simulink model "FINAL"  (R2021a)
settings: Solver=ode4  StartTime=0.0  StopTime=tfinal*6.5  FixedStep=dt  RelTol=1e-3
undefined symbols (not defined in the file): A, A_Lat, B, B0, B_Lat, bsi0, C, C_Lat, D, D_Lateral, Der, dt, Earth, g, K, K_D, K_Dh, K_Du, K_PI, K_PIh, K_PIu, m, mg0, p0, P_Du, P_PI, P_PIu, phi0, q0, r0, s0, sigbuilder_block, theta0, u0, v0, w0, WGS84, y, Z_Du, Z_PI, Z_PIu
libraries: simulink_extras x23, cstblocks x6, aerolibfltsims x2, shared6dof x1, aerolibtransform2 x1, aerolibasang x1, dspsigops x1
settings Model: Creator=bahbo  LastModifiedBy=bahbo

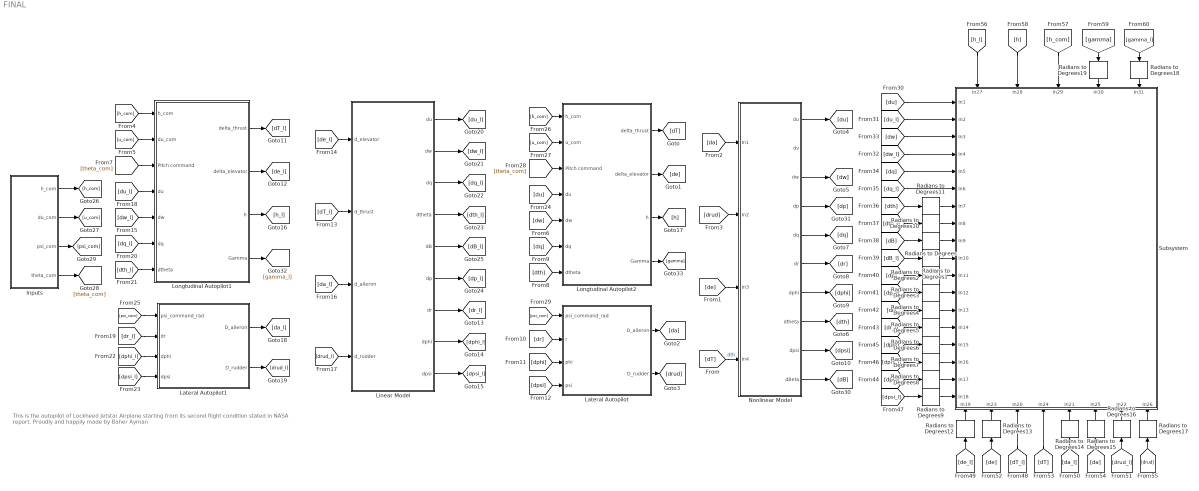
== system FINAL ==
  note: This is the autopilot of Lockheed Jetstar Airplane starting from its second flight condition stated in NASA report.
      | Proudly and happily made by Baher Ayman
  Inputs : Subsystem
  Lateral Autopilot : Subsystem
  Lateral Autopilot1 : Subsystem
  Linear Model : Subsystem
  Longtudinal Autopilot1 : Subsystem
  Longtudinal Autopilot2 : Subsystem
  Nonlinear Model : Subsystem
  Radians to Degrees{,1..19} (20 alike) : simulink_extras/Transformations/Radians to Degrees
  Subsystem : Subsystem
      settings: PortSchema="{\"entries\":[{\"content\":{\"sides\":[{\"content\":{\"connectorIds\":[\"In1\",\"In2\",\"In3\",\"In4\",\"In5\",\"In6\",\"In7\",\"In8\",\"In9\",\"In10\",\"In11\",\"In12\",\"In13\",\"In14\",\"In15\",\"In16\",\"In17\",\"In18\"]},\"type\":\"ConnectorPlacement.EquallySpacedRectSide\",\"uuid\":\"e5837911-82e8-4f0c-8622-00ee6713ee26\"},{\"content\":{\"connectorIds\":[],\"side\":\"RIGHT\"},\"type\":\"ConnectorPlacement.EquallySpacedRectSide\",\"uuid\":\"5100fd71-1e10-46a1-997f-a1a366e3eb4d\"},{\"content\":{\"connectorIds\":[\"In19\",\"In20\",\"In21\",\"In22\",\"In23\"],\"side\":\"TOP\"},\"type\":\"ConnectorPlacement.EquallySpacedRectSide\",\"uuid\":\"f99c9fc8-e14b-4975-9fcd-b405dd621b26\"},{\"content\":{\"connectorIds\":[\"In24\",\"In25\",\"In26\",\"In27\",\"In28\",\"In29\",\"In30\",\"In31\"],\"side\":\"BOTTOM\"},\"type\":\"ConnectorPlacement.EquallySpacedRectSide\",\"uuid\":\"bb89a20a-82c0-43e7-b765-f41e6636c457\"}]},\"type\":\"ConnectorPlacement.EquallySpacedConnector\",\"uuid\":\"6d5563cc-839d-4a7b-b6e3-37355380fa60\"}],\"packageUris\":[\"http://schema.mathworks.com/mf0/Connector/R2020b\"],\"version\":\"1.0\"}"
  wires:
  [de] -> Nonlinear Model/3(In3)
  Longtudinal Autopilot2/2(delta_elevator) -> [de]
  Lateral Autopilot/2(D_rudder) -> [drud]
  [drud] -> Nonlinear Model/2(In2)
  Nonlinear Model/5(dq) -> [dq]
  Nonlinear Model/8(dtheta) -> [dth]
  [dpsi] -> Lateral Autopilot/4(psi)
  Nonlinear Model/6(dr) -> [dr]
  [dq] -> Longtudinal Autopilot2/6(dq)
  Nonlinear Model/9(dpsi) -> [dpsi]
  Nonlinear Model/1(du) -> [du]
  Lateral Autopilot/1(D_aileron) -> [da]
  Nonlinear Model/7(dphi) -> [dphi]
  [dT] -> Nonlinear Model/4(In4)  "dth"
  [da] -> Nonlinear Model/1(In1)
  Longtudinal Autopilot2/1(delta_thrust) -> [dT]
  Nonlinear Model/3(dw) -> [dw]
  [dphi] -> Lateral Autopilot/3(phi)
  [dth] -> Longtudinal Autopilot2/7(dtheta)
  [dr] -> Lateral Autopilot/2(r)
  Linear Model/1(du) -> [du_l]
  Linear Model/7(dr) -> [dr_l]
  Linear Model/3(dq) -> [dq_l]
  Longtudinal Autopilot1/3(h) -> [h_l]
  [dpsi_l] -> Lateral Autopilot1/4(dpsi)
  [dw_l] -> Longtudinal Autopilot1/5(dw)
  Linear Model/9(dpsi) -> [dpsi_l]
  Longtudinal Autopilot1/1(delta_thrust) -> [dT_l]
  Lateral Autopilot1/2(D_rudder) -> [drud_l]
  [dphi_l] -> Lateral Autopilot1/3(dphi)
  [drud_l] -> Linear Model/4(d_rudder)
  [dq_l] -> Longtudinal Autopilot1/6(dq)
  [de_l] -> Linear Model/1(d_elevator)
  [du_l] -> Longtudinal Autopilot1/4(du)
  Linear Model/5(dB) -> [dB_l]
  Linear Model/6(dp) -> [dp_l]
  [da_l] -> Linear Model/3(d_aileron)
  Longtudinal Autopilot1/2(delta_elevator) -> [de_l]
  Lateral Autopilot1/1(D_aileron) -> [da_l]
  Linear Model/4(dtheta) -> [dth_l]
  [dT_l] -> Linear Model/2(d_thrust)
  [dr_l] -> Lateral Autopilot1/2(dr)
  [dth_l] -> Longtudinal Autopilot1/7(dtheta)
  Linear Model/8(dphi) -> [dphi_l]
  Linear Model/2(dw) -> [dw_l]
  [du] -> Longtudinal Autopilot2/4(du)
  [dw] -> Longtudinal Autopilot2/5(dw)
  Inputs/2(du_com) -> [u_com]
  Inputs/4(theta_com) -> [theta_com]
  Inputs/1(h_com) -> [h_com]
  Inputs/3(psi_com) -> [psi_com]
  [h_com] -> Longtudinal Autopilot1/1(h_com)
  [u_com] -> Longtudinal Autopilot1/2(du_com)
  [theta_com] -> Longtudinal Autopilot1/3(Pitch command)
  [psi_com] -> Lateral Autopilot1/1(psi_command_rad)
  [h_com] -> Longtudinal Autopilot2/1(h_com)
  [u_com] -> Longtudinal Autopilot2/2(u_com)
  [theta_com] -> Longtudinal Autopilot2/3(Pitch command)
  [psi_com] -> Lateral Autopilot/1(psi_command_rad)
  Nonlinear Model/10(dBeta) -> [dB]
  [du] -> Subsystem/1(In1)
  [du_l] -> Subsystem/2(In2)
  [dw_l] -> Subsystem/4(In4)
  [dw] -> Subsystem/3(In3)
  [dq] -> Subsystem/5(In5)
  [dq_l] -> Subsystem/6(In6)
  Nonlinear Model/4(dp) -> [dp]
  [dT_l] -> Subsystem/26(In20)
  [dT] -> Subsystem/27(In24)
  Longtudinal Autopilot2/3(h) -> [h]
  [h_l] -> Subsystem/19(In27)
  [h] -> Subsystem/20(In28)
  [h_com] -> Subsystem/21(In29)
  Radians to Degrees9/1 -> Subsystem/18(In18)
  [dpsi_l] -> Radians to Degrees9/1
  [dpsi] -> Radians to Degrees8/1
  Radians to Degrees8/1 -> Subsystem/17(In17)
  [dphi_l] -> Radians to Degrees7/1
  Radians to Degrees7/1 -> Subsystem/16(In16)
  [dphi] -> Radians to Degrees6/1
  Radians to Degrees6/1 -> Subsystem/15(In15)
  [dr_l] -> Radians to Degrees5/1
  Radians to Degrees5/1 -> Subsystem/14(In14)
  [dr] -> Radians to Degrees4/1
  Radians to Degrees4/1 -> Subsystem/13(In13)
  [dp_l] -> Radians to Degrees3/1
  Radians to Degrees3/1 -> Subsystem/12(In12)
  [dp] -> Radians to Degrees2/1
  Radians to Degrees2/1 -> Subsystem/11(In11)
  [dB_l] -> Radians to Degrees1/1
  Radians to Degrees1/1 -> Subsystem/10(In10)
  [dB] -> Radians to Degrees/1
  Radians to Degrees/1 -> Subsystem/9(In9)
  [dth] -> Radians to Degrees11/1
  Radians to Degrees11/1 -> Subsystem/7(In7)
  [dth_l] -> Radians to Degrees10/1
  Radians to Degrees10/1 -> Subsystem/8(In8)
  Radians to Degrees16/1 -> Subsystem/30(In22)
  [drud_l] -> Radians to Degrees16/1
  [drud] -> Radians to Degrees17/1
  Radians to Degrees17/1 -> Subsystem/31(In26)
  [da] -> Radians to Degrees15/1
  Radians to Degrees15/1 -> Subsystem/29(In25)
  [da_l] -> Radians to Degrees14/1
  Radians to Degrees14/1 -> Subsystem/28(In21)
  [de] -> Radians to Degrees13/1
  Radians to Degrees13/1 -> Subsystem/25(In23)
  [de_l] -> Radians to Degrees12/1
  Radians to Degrees12/1 -> Subsystem/24(In19)
  Longtudinal Autopilot1/4(Gamma) -> [gamma_l]
  Longtudinal Autopilot2/4(Gamma) -> [gamma]
  [gamma] -> Radians to Degrees19/1
  [gamma_l] -> Radians to Degrees18/1
  Radians to Degrees18/1 -> Subsystem/23(In31)
  Radians to Degrees19/1 -> Subsystem/22(In30)

== system FINAL/Inputs ==
  Constant : Constant  Commented=on  Value=12
  Degrees to Radians : simulink_extras/Transformations/Degrees to Radians  Commented=on
  Inputs Signals : Subsystem  Tag=STV Subsys  LoadFcn=sigbuilder_block('load');  StartFcn=sigbuilder_block('start');  StopFcn=sigbuilder_block('stop');  ClipboardFcn=sigbuilder_block('clipboard');  mask(Sigbuilder block){tuvar=[0:10]}
      mask help: Simulink:masks:SigbuilderBlock_MD
      mask init:
      | if ~strcmp(get_param(bdroot(gcbh),'SimulationStatus'),'stopped') tuvar = sigbuilder_block('maskInit'); end
      settings: CopyFcn=sigbuilder_block('copy');  DeleteFcn=sigbuilder_block('delete');  ModelCloseFcn=sigbuilder_block('modelClose');  PreSaveFcn=sigbuilder_block('preSave');  PauseFcn=sigbuilder_block('pause');  ContinueFcn=sigbuilder_block('continue');  NameChangeFcn=sigbuilder_block('namechange');  OpenFcn=sigbuilder_block('open',[6 33 1012.5 444 ]);  CloseFcn=sigbuilder_block('close');
      mask Display: plot(0, 0, 100, 100,[2, 2, 32, 32, 2], [68, 8, 8, 68, 68],[32, 2], [38, 38], [32, 19, 2],[53, 60, 44], [32, 17, 17, 2],[16, 16, 31, 31]);txt = getActiveGroup(gcbh);text(2, 100, txt,'verticalAlignment', 'top');
  h_com : Outport
  du_com : Outport  Port=2
  psi_com : Outport  Port=3
  theta_com : Outport  Port=4
  wires:
  Inputs Signals/3(Velocity Com.) -> du_com/1
  Constant/1 -> Degrees to Radians/1
  Degrees to Radians/1 -> theta_com/1
  Inputs Signals/1(Altitude Command) -> h_com/1
  Inputs Signals/2(Psi Command) -> psi_com/1

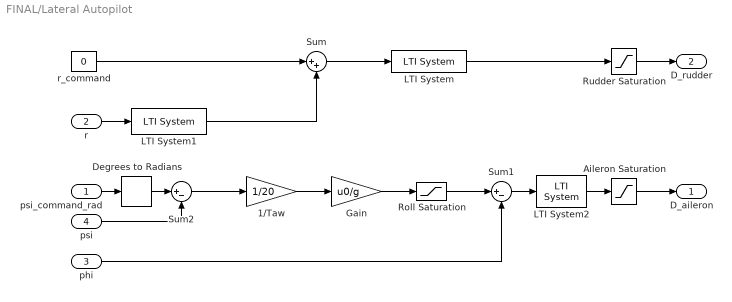
== system FINAL/Lateral Autopilot ==
  psi_command_rad : Inport
  r : Inport  Port=2
  phi : Inport  Port=3
  psi : Inport  Port=4
  1/Taw : Gain  Gain=1/20
  Aileron Saturation : Saturate  UpperLimit=50*pi/180  LowerLimit=-50*pi/180
  Degrees to Radians : simulink_extras/Transformations/Degrees to Radians
  Gain : Gain  Gain=u0/g
  LTI System : cstblocks/LTI System  sys=servo  IC=[]
  LTI System1 : cstblocks/LTI System  sys=yaw_damper  IC=[]
  LTI System2 : cstblocks/LTI System  sys=roll_ctrl  IC=[]
  Roll Saturation : Saturate  UpperLimit=30*pi/180  LowerLimit=-30*pi/180
  Rudder Saturation : Saturate  UpperLimit=15*pi/180  LowerLimit=-15*pi/180
  Sum : Sum  Inputs=|++
  Sum1 : Sum  Inputs=|+-
  Sum2 : Sum  Inputs=|+-
  r_command : Constant  Value=0
  D_aileron : Outport
  D_rudder : Outport  Port=2
  wires:
  Sum2/1 -> 1/Taw/1
  Sum/1 -> LTI System/1
  r/1 -> LTI System1/1
  Rudder Saturation/1 -> D_rudder/1
  Roll Saturation/1 -> Sum1/1
  Aileron Saturation/1 -> D_aileron/1
  r_command/1 -> Sum/1
  phi/1 -> Sum1/2
  psi/1 -> Sum2/2
  LTI System1/1 -> Sum/2
  LTI System/1 -> Rudder Saturation/1
  Sum1/1 -> LTI System2/1
  1/Taw/1 -> Gain/1
  Gain/1 -> Roll Saturation/1
  LTI System2/1 -> Aileron Saturation/1
  psi_command_rad/1 -> Degrees to Radians/1
  Degrees to Radians/1 -> Sum2/1

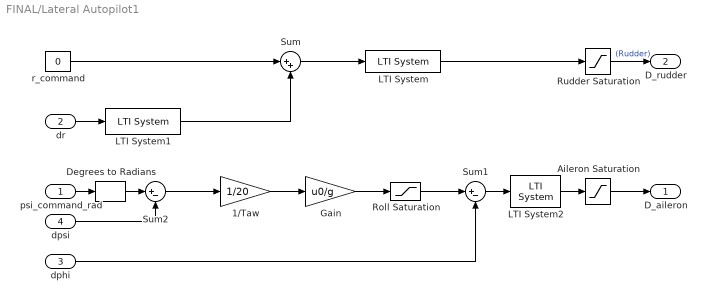
== system FINAL/Lateral Autopilot1 ==
  psi_command_rad : Inport
  dr : Inport  Port=2
  dphi : Inport  Port=3
  dpsi : Inport  Port=4
  1/Taw : Gain  Gain=1/20
  Aileron Saturation : Saturate  UpperLimit=50*pi/180  LowerLimit=-50*pi/180
  Degrees to Radians : simulink_extras/Transformations/Degrees to Radians
  Gain : Gain  Gain=u0/g
  LTI System : cstblocks/LTI System  sys=servo  IC=[]
  LTI System1 : cstblocks/LTI System  sys=yaw_damper  IC=[]
  LTI System2 : cstblocks/LTI System  sys=roll_ctrl  IC=[]
  Roll Saturation : Saturate  UpperLimit=30*pi/180  LowerLimit=-30*pi/180
  Rudder Saturation : Saturate  UpperLimit=15*pi/180  LowerLimit=-15*pi/180
  Sum : Sum  Inputs=|++
  Sum1 : Sum  Inputs=|+-
  Sum2 : Sum  Inputs=|+-
  r_command : Constant  Value=0
  D_aileron : Outport
  D_rudder : Outport  Port=2
  wires:
  Sum2/1 -> 1/Taw/1
  Sum/1 -> LTI System/1
  dr/1 -> LTI System1/1
  Rudder Saturation/1 -> D_rudder/1  "(Rudder)"
  Roll Saturation/1 -> Sum1/1
  Aileron Saturation/1 -> D_aileron/1
  r_command/1 -> Sum/1
  dphi/1 -> Sum1/2
  dpsi/1 -> Sum2/2
  LTI System1/1 -> Sum/2
  LTI System/1 -> Rudder Saturation/1
  Sum1/1 -> LTI System2/1
  1/Taw/1 -> Gain/1
  Gain/1 -> Roll Saturation/1
  LTI System2/1 -> Aileron Saturation/1
  psi_command_rad/1 -> Degrees to Radians/1
  Degrees to Radians/1 -> Sum2/1

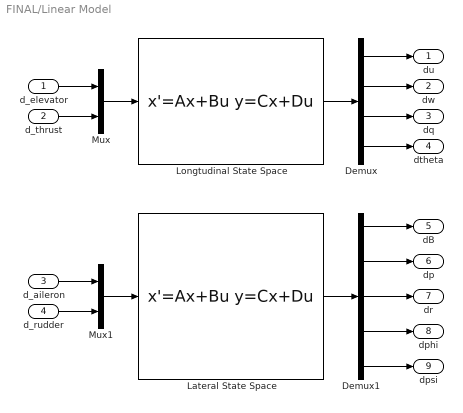
== system FINAL/Linear Model ==
  d_elevator : Inport
  d_thrust : Inport  Port=2
  d_aileron : Inport  Port=3
  d_rudder : Inport  Port=4
  Demux : Demux
  Demux1 : Demux  Outputs=5
  Lateral State Space : StateSpace  A=A_Lat  B=B_Lat  C=C_Lat  D=D_Lateral  InitialCondition=0
  Longtudinal State Space : StateSpace  A=A  B=B  C=C  D=D  InitialCondition=0
  Mux : Mux  Inputs=2
  Mux1 : Mux  Inputs=2
  du : Outport
  dw : Outport  Port=2
  dq : Outport  Port=3
  dtheta : Outport  Port=4
  dB : Outport  Port=5
  dp : Outport  Port=6
  dr : Outport  Port=7
  dphi : Outport  Port=8
  dpsi : Outport  Port=9
  wires:
  Demux/3 -> dq/1
  Lateral State Space/1 -> Demux1/1
  Demux1/4 -> dphi/1
  d_elevator/1 -> Mux/1
  Demux/4 -> dtheta/1
  Mux/1 -> Longtudinal State Space/1
  Mux1/1 -> Lateral State Space/1
  d_thrust/1 -> Mux/2
  Demux1/5 -> dpsi/1
  Demux1/1 -> dB/1
  Demux1/2 -> dp/1
  Demux/2 -> dw/1
  d_aileron/1 -> Mux1/1
  Demux/1 -> du/1
  Demux1/3 -> dr/1
  Longtudinal State Space/1 -> Demux/1
  d_rudder/1 -> Mux1/2

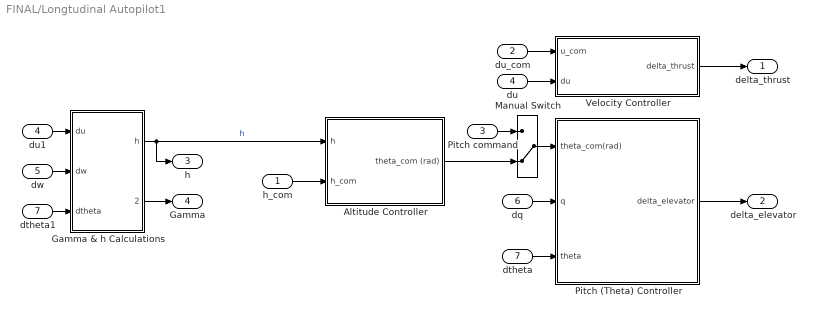
== system FINAL/Longtudinal Autopilot1 ==
  h_com : Inport
  du_com : Inport  Port=2
  Pitch command : Inport  Port=3
  du : Inport  Port=4
  dw : Inport  Port=5
  dq : Inport  Port=6
  dtheta : Inport  Port=7
  Altitude Controller : Subsystem
  Gamma & h Calculations : Subsystem
  Manual Switch : ManualSwitch  CurrentSetting=0
  Pitch (Theta) Controller : Subsystem
  Velocity Controller : Subsystem
  dtheta1 : InportShadow  Port=7
  du1 : InportShadow  Port=4
  delta_thrust : Outport
  delta_elevator : Outport  Port=2
  h : Outport  Port=3
  Gamma : Outport  Port=4
  wires:
  du/1 -> Velocity Controller/2(du)
  Velocity Controller/1(delta_thrust) -> delta_thrust/1
  dtheta/1 -> Pitch (Theta) Controller/3(theta)
  h_com/1 -> Altitude Controller/2(h_com)
  du_com/1 -> Velocity Controller/1(u_com)
  Pitch (Theta) Controller/1(delta_elevator) -> delta_elevator/1
  dq/1 -> Pitch (Theta) Controller/2(q)
  Altitude Controller/1(theta_com (rad)) -> Manual Switch/2
  Manual Switch/1 -> Pitch (Theta) Controller/1(theta_com(rad))
  Pitch command/1 -> Manual Switch/1
  du1/1 -> Gamma & h Calculations/1(du)
  dtheta1/1 -> Gamma & h Calculations/3(dtheta)
  Gamma & h Calculations/1(h) -> Altitude Controller/1(h), h/1  "h"
  dw/1 -> Gamma & h Calculations/2(dw)
  Gamma & h Calculations/2(gamma) -> Gamma/1

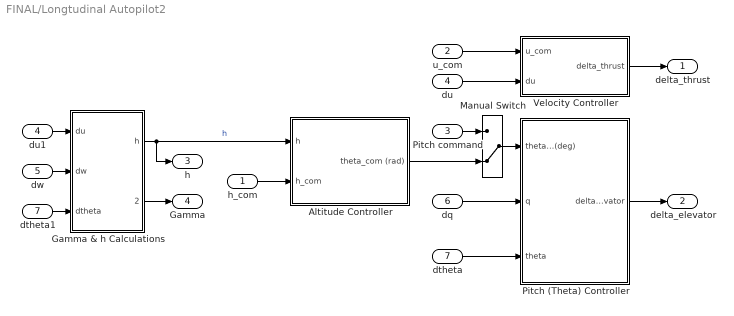
== system FINAL/Longtudinal Autopilot2 ==
  h_com : Inport
  u_com : Inport  Port=2
  Pitch command : Inport  Port=3
  du : Inport  Port=4
  dw : Inport  Port=5
  dq : Inport  Port=6
  dtheta : Inport  Port=7
  Altitude Controller : Subsystem
  Gamma & h Calculations : Subsystem
  Manual Switch : ManualSwitch  CurrentSetting=0
  Pitch (Theta) Controller : Subsystem
  Velocity Controller : Subsystem
  dtheta1 : InportShadow  Port=7
  du1 : InportShadow  Port=4
  delta_thrust : Outport
  delta_elevator : Outport  Port=2
  h : Outport  Port=3
  Gamma : Outport  Port=4
  wires:
  du/1 -> Velocity Controller/2(du)
  Velocity Controller/1(delta_thrust) -> delta_thrust/1
  dtheta/1 -> Pitch (Theta) Controller/3(theta)
  h_com/1 -> Altitude Controller/2(h_com)
  u_com/1 -> Velocity Controller/1(u_com)
  Pitch (Theta) Controller/1(delta_elevator) -> delta_elevator/1
  dq/1 -> Pitch (Theta) Controller/2(q)
  Altitude Controller/1(theta_com (rad)) -> Manual Switch/2
  Manual Switch/1 -> Pitch (Theta) Controller/1(theta_com(deg))
  Pitch command/1 -> Manual Switch/1
  du1/1 -> Gamma & h Calculations/1(du)
  dtheta1/1 -> Gamma & h Calculations/3(dtheta)
  Gamma & h Calculations/1(h) -> Altitude Controller/1(h), h/1  "h"
  dw/1 -> Gamma & h Calculations/2(dw)
  Gamma & h Calculations/2(gamma) -> Gamma/1

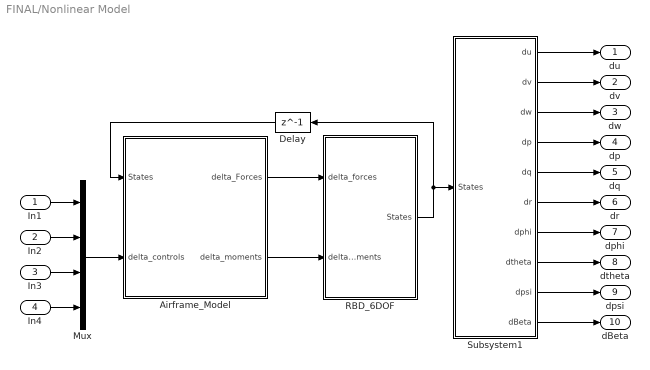
== system FINAL/Nonlinear Model ==
  In1 : Inport
  In2 : Inport  Port=2
  In3 : Inport  Port=3
  In4 : Inport  Port=4
  Airframe_Model : Subsystem
  Delay : Delay  DelayLength=1  InitialCondition=K
  Mux : Mux
  RBD_6DOF : Subsystem
  Subsystem1 : Subsystem
  du : Outport
  dv : Outport  Port=2
  dw : Outport  Port=3
  dp : Outport  Port=4
  dq : Outport  Port=5
  dr : Outport  Port=6
  dphi : Outport  Port=7
  dtheta : Outport  Port=8
  dpsi : Outport  Port=9
  dBeta : Outport  Port=10
  wires:
  RBD_6DOF/1(States) -> Delay/1, Subsystem1/1(States)
  Airframe_Model/2(delta_moments) -> RBD_6DOF/2(delta_moments)
  Subsystem1/4(dp) -> dp/1
  Delay/1 -> Airframe_Model/1(States)
  Subsystem1/7(dphi) -> dphi/1
  Mux/1 -> Airframe_Model/2(delta_controls)
  In2/1 -> Mux/2
  Airframe_Model/1(delta_Forces) -> RBD_6DOF/1(delta_forces)
  Subsystem1/8(dtheta) -> dtheta/1
  In1/1 -> Mux/1
  Subsystem1/6(dr) -> dr/1
  Subsystem1/5(dq) -> dq/1
  In3/1 -> Mux/3
  Subsystem1/1(du) -> du/1
  In4/1 -> Mux/4
  Subsystem1/3(dw) -> dw/1
  Subsystem1/10(dBeta) -> dBeta/1
  Subsystem1/9(dpsi) -> dpsi/1
  Subsystem1/2(dv) -> dv/1

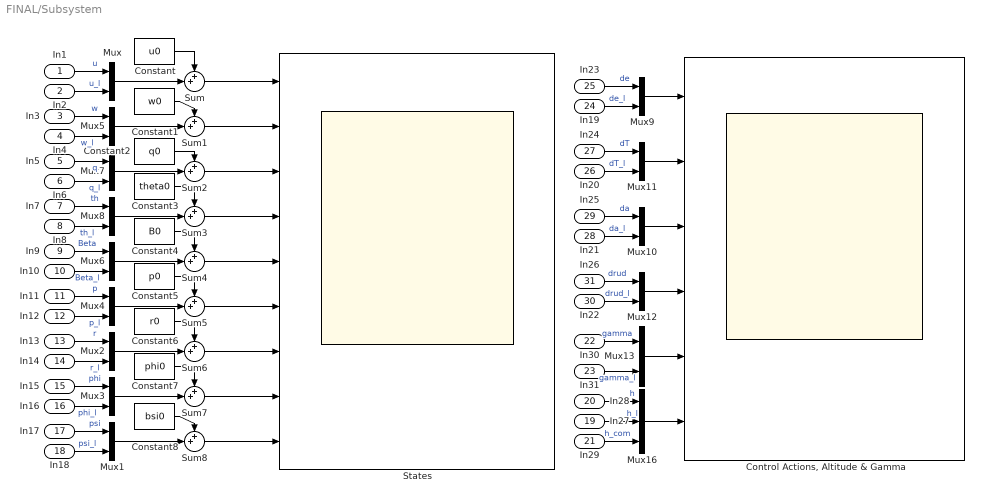
== system FINAL/Subsystem ==
  In1 : Inport
  In2 : Inport  Port=2
  In3 : Inport  Port=3
  In4 : Inport  Port=4
  In5 : Inport  Port=5
  In6 : Inport  Port=6
  In7 : Inport  Port=7
  In8 : Inport  Port=8
  In9 : Inport  Port=9
  In10 : Inport  Port=10
  In11 : Inport  Port=11
  In12 : Inport  Port=12
  In13 : Inport  Port=13
  In14 : Inport  Port=14
  In15 : Inport  Port=15
  In16 : Inport  Port=16
  In17 : Inport  Port=17
  In18 : Inport  Port=18
  In27 : Inport  Port=19
  In28 : Inport  Port=20
  In29 : Inport  Port=21
  In30 : Inport  Port=22
  In31 : Inport  Port=23
  In19 : Inport  Port=24
  In23 : Inport  Port=25
  In20 : Inport  Port=26
  In24 : Inport  Port=27
  In21 : Inport  Port=28
  In25 : Inport  Port=29
  In22 : Inport  Port=30
  In26 : Inport  Port=31
  Constant : Constant  Value=u0
  Constant1 : Constant  Value=w0
  Constant2 : Constant  Value=q0
  Constant3 : Constant  Value=theta0
  Constant4 : Constant  Value=B0
  Constant5 : Constant  Value=p0
  Constant6 : Constant  Value=r0
  Constant7 : Constant  Value=phi0
  Constant8 : Constant  Value=bsi0
  "Control Actions, Altitude & Gamma" : Scope  NumInputPorts=6
  Mux{,1..13} (14 alike) : Mux  Inputs=2
  Mux16 : Mux  Inputs=3
  States : Scope  NumInputPorts=9
  Sum{,1..8} (9 alike) : Sum  Inputs=++|
  wires:
  Mux9/1 -> "Control Actions, Altitude & Gamma"/1
  Mux10/1 -> "Control Actions, Altitude & Gamma"/3
  Mux11/1 -> "Control Actions, Altitude & Gamma"/2
  Mux12/1 -> "Control Actions, Altitude & Gamma"/4
  Mux16/1 -> "Control Actions, Altitude & Gamma"/6
  In1/1 -> Mux/1  "u"
  In3/1 -> Mux5/1  "w"
  In4/1 -> Mux5/2  "w_l"
  In5/1 -> Mux7/1  "q"
  In6/1 -> Mux7/2  "q_l"
  In7/1 -> Mux8/1  "th"
  In8/1 -> Mux8/2  "th_l"
  In9/1 -> Mux6/1  "Beta"
  In10/1 -> Mux6/2  "Beta_l"
  In11/1 -> Mux4/1  "p"
  In12/1 -> Mux4/2  "p_l"
  In13/1 -> Mux2/1  "r"
  In14/1 -> Mux2/2  "r_l"
  In15/1 -> Mux3/1  "phi"
  In16/1 -> Mux3/2  "phi_l"
  In17/1 -> Mux1/1  "psi"
  In18/1 -> Mux1/2  "psi_l"
  In2/1 -> Mux/2  "u_l"
  In19/1 -> Mux9/2  "de_l"
  In20/1 -> Mux11/2  "dT_l"
  In21/1 -> Mux10/2  "da_l"
  In22/1 -> Mux12/2  "drud_l"
  In23/1 -> Mux9/1  "de"
  In24/1 -> Mux11/1  "dT"
  In25/1 -> Mux10/1  "da"
  In26/1 -> Mux12/1  "drud"
  In27/1 -> Mux16/2  "h_l"
  In28/1 -> Mux16/1  "h"
  In29/1 -> Mux16/3  "h_com"
  In30/1 -> Mux13/1  "gamma"
  In31/1 -> Mux13/2  "gamma_l"
  Mux13/1 -> "Control Actions, Altitude & Gamma"/5
  Sum/1 -> States/1
  Mux/1 -> Sum/2
  Constant/1 -> Sum/1
  Constant1/1 -> Sum1/1
  Mux5/1 -> Sum1/2
  Sum1/1 -> States/2
  Constant2/1 -> Sum2/1
  Mux7/1 -> Sum2/2
  Sum2/1 -> States/3
  Constant3/1 -> Sum3/1
  Mux8/1 -> Sum3/2
  Sum3/1 -> States/4
  Constant4/1 -> Sum4/1
  Mux6/1 -> Sum4/2
  Sum4/1 -> States/5
  Constant5/1 -> Sum5/1
  Mux4/1 -> Sum5/2
  Sum5/1 -> States/6
  Constant6/1 -> Sum6/1
  Mux2/1 -> Sum6/2
  Sum6/1 -> States/7
  Constant7/1 -> Sum7/1
  Mux3/1 -> Sum7/2
  Sum7/1 -> States/8
  Constant8/1 -> Sum8/1
  Mux1/1 -> Sum8/2
  Sum8/1 -> States/9

== system FINAL/Inputs/Inputs Signals ==
  Demux : Demux  Tag=STV Demux  Outputs=3
      settings: DisplayOption=none
  FromWs : FromWorkspace  Tag=STV FromWs  VariableName=tuvar
      SigBuilderData=|
      | common.afterFinalStr = 'Extrapolate'
      | common.sampleTime = 0
      | dataSet.timeRange = [0 1300]
      | dataSet.name = 'Group 1'
      | sbobj.Groups.Name = 'Group 1'
      | sbobj.Groups.Signals(1).Name = 'Altitude Command'
      | sbobj.Groups.Signals(1).XData = [0 400 520 760 760 880 1284 1300]
      | sbobj.Groups.Signals(1).YData = [0 10000 10000 10000 10100 10100 0 0]
      | sbobj.Groups.Signals(2).Name = 'Psi Command'
      | sbobj.Groups.Signals(2).XData = [0 520 520 760 760 1300]
      | sbobj.Groups.Signals(2).YData = [0 0 360 360 390 390]
      | sbobj.Groups.Signals(3).Name = 'Velocity Com.'
      | sbobj.Groups.Signals(3).XData = [0 400 1000 1284 1300]
      | sbobj.Groups.Signals(3).YData = [0 400 400 0 0]
      | sbobj.Groups.TimeRange = [0 1300]
  Altitude Command : Outport  Tag=STV Outport
  Psi Command : Outport  Tag=STV Outport  Port=2
  Velocity Com. : Outport  Tag=STV Outport  Port=3
  wires:
  FromWs/1 -> Demux/1
  Demux/1 -> Altitude Command/1
  Demux/2 -> Psi Command/1
  Demux/3 -> Velocity Com./1

== system FINAL/Longtudinal Autopilot1/Altitude Controller ==
  note: Altitude Controller
  h : Inport
  h_com : Inport  Port=2
  Differentiator : Derivative
  Kd : Gain  Gain=K_Dh
  Kp : Gain  Gain=K_PIh
  Sum : Sum  Inputs=|+-
  Sum1 : Sum  Inputs=|+-
  theta_com (rad) : Outport
  wires:
  Sum/1 -> theta_com (rad)/1
  Sum1/1 -> Kp/1
  Kd/1 -> Sum/2
  h_com/1 -> Sum1/1
  Kp/1 -> Sum/1
  Differentiator/1 -> Kd/1
  h/1 -> Sum1/2, Differentiator/1

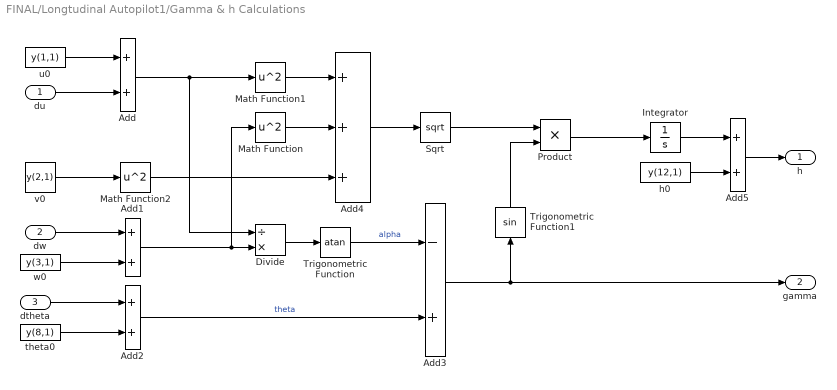
== system FINAL/Longtudinal Autopilot1/Gamma & h Calculations ==
  du : Inport
  dw : Inport  Port=2
  dtheta : Inport  Port=3
  Add{,1..2,5} (4 alike) : Sum
  Add3 : Sum  Inputs=-+
  Add4 : Sum  Inputs=+++
  Divide : Product  Inputs=/*
  Integrator : Integrator
  Math Function : Math  Operator=square  SignedPower=on  SaturateOnIntegerOverflow=on
  Math Function1 : Math  Operator=square  SignedPower=on  SaturateOnIntegerOverflow=on
  Math Function2 : Math  Operator=square  SignedPower=on  SaturateOnIntegerOverflow=on
  Product : Product
  Sqrt : Sqrt  SaturateOnIntegerOverflow=on
  Trigonometric Function : Trigonometry  Operator=atan
  Trigonometric Function1 : Trigonometry
  h0 : Constant  Value=y(12,1)
  theta0 : Constant  Value=y(8,1)
  u0 : Constant  Value=y(1,1)
  v0 : Constant  Value=y(2,1)
  w0 : Constant  Value=y(3,1)
  h : Outport
  gamma : Outport  Port=2
  wires:
  Integrator/1 -> Add5/1
  Product/1 -> Integrator/1
  h0/1 -> Add5/2
  Divide/1 -> Trigonometric Function/1
  Math Function1/1 -> Add4/1
  Add5/1 -> h/1
  Trigonometric Function1/1 -> Product/2
  Add3/1 -> gamma/1, Trigonometric Function1/1
  Add4/1 -> Sqrt/1
  Trigonometric Function/1 -> Add3/1  "alpha"
  Math Function/1 -> Add4/2
  Sqrt/1 -> Product/1
  Math Function2/1 -> Add4/3
  v0/1 -> Math Function2/1
  Add/1 -> Math Function1/1, Divide/1
  u0/1 -> Add/1
  du/1 -> Add/2
  w0/1 -> Add1/2
  dw/1 -> Add1/1
  Add1/1 -> Math Function/1, Divide/2
  dtheta/1 -> Add2/1
  theta0/1 -> Add2/2
  Add2/1 -> Add3/2  "theta"

== system FINAL/Longtudinal Autopilot1/Pitch (Theta) Controller ==
  note: Pitch Controller
  theta_com(rad) : Inport
  q : Inport  Port=2
  theta : Inport  Port=3
  Elevator Saturation : Saturate  UpperLimit=25*pi/180  LowerLimit=-25*pi/180
  Kd : Gain  Gain=K_D
  Sum : Sum  Inputs=|+-
  Sum1 : Sum  Inputs=|+-
  Zero-Pole : ZeroPole  Zeros=[Z_PI]  Poles=[P_PI]  Gain=[K_PI]
  servo : TransferFcn  Numerator=[-10]  Denominator=[1 10]
  delta_elevator : Outport
  wires:
  q/1 -> Kd/1
  Zero-Pole/1 -> Sum/1
  Sum/1 -> servo/1
  theta_com(rad)/1 -> Sum1/1
  Kd/1 -> Sum/2
  theta/1 -> Sum1/2
  servo/1 -> Elevator Saturation/1
  Sum1/1 -> Zero-Pole/1
  Elevator Saturation/1 -> delta_elevator/1

== system FINAL/Longtudinal Autopilot1/Velocity Controller ==
  note: Velocity Controller
  u_com : Inport
  du : Inport  Port=2
  Engine Saturation : Saturate  UpperLimit=3*3700  LowerLimit=-1500
  Sum : Sum  Inputs=|+-
  Sum1 : Sum  Inputs=|+-
  Zero-Pole : ZeroPole  Zeros=[Z_Du]  Poles=[P_Du]  Gain=[K_Du]
  Zero-Pole1 : ZeroPole  Zeros=[Z_PIu]  Poles=[P_PIu]  Gain=[K_PIu]
  engine_timelag : TransferFcn  Numerator=[0.1]  Denominator=[1 0.1]
  servo : TransferFcn  Numerator=[10]  Denominator=[1 10]
  delta_thrust : Outport
  wires:
  u_com/1 -> Sum1/1
  Sum/1 -> servo/1
  servo/1 -> engine_timelag/1
  du/1 -> Sum1/2, Zero-Pole/1
  engine_timelag/1 -> Engine Saturation/1
  Zero-Pole/1 -> Sum/2
  Sum1/1 -> Zero-Pole1/1
  Zero-Pole1/1 -> Sum/1
  Engine Saturation/1 -> delta_thrust/1

== system FINAL/Longtudinal Autopilot2/Altitude Controller ==
  note: Altitude Controller
  h : Inport
  h_com : Inport  Port=2
  Differentiator : Derivative
  Kd : Gain  Gain=K_Dh
  Kp : Gain  Gain=K_PIh
  Sum : Sum  Inputs=|+-
  Sum1 : Sum  Inputs=|+-
  theta_com (rad) : Outport
  wires:
  Sum/1 -> theta_com (rad)/1
  Sum1/1 -> Kp/1
  Kd/1 -> Sum/2
  h_com/1 -> Sum1/1
  Kp/1 -> Sum/1
  Differentiator/1 -> Kd/1
  h/1 -> Sum1/2, Differentiator/1

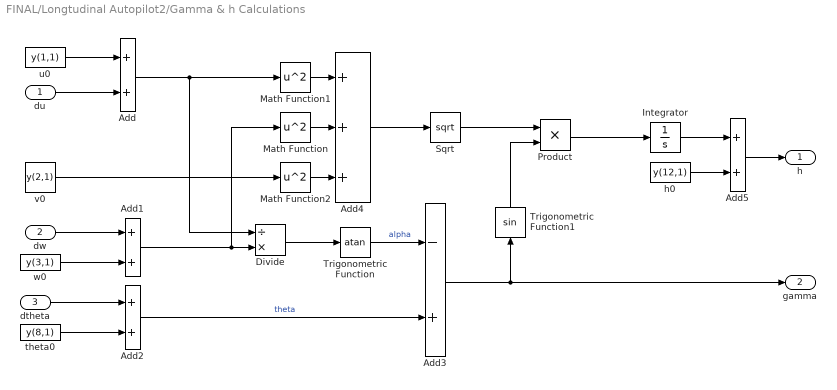
== system FINAL/Longtudinal Autopilot2/Gamma & h Calculations ==
  du : Inport
  dw : Inport  Port=2
  dtheta : Inport  Port=3
  Add{,1..2,5} (4 alike) : Sum
  Add3 : Sum  Inputs=-+
  Add4 : Sum  Inputs=+++
  Divide : Product  Inputs=/*
  Integrator : Integrator
  Math Function : Math  Operator=square  SignedPower=on  SaturateOnIntegerOverflow=on
  Math Function1 : Math  Operator=square  SignedPower=on  SaturateOnIntegerOverflow=on
  Math Function2 : Math  Operator=square  SignedPower=on  SaturateOnIntegerOverflow=on
  Product : Product
  Sqrt : Sqrt  SaturateOnIntegerOverflow=on
  Trigonometric Function : Trigonometry  Operator=atan
  Trigonometric Function1 : Trigonometry
  h0 : Constant  Value=y(12,1)
  theta0 : Constant  Value=y(8,1)
  u0 : Constant  Value=y(1,1)
  v0 : Constant  Value=y(2,1)
  w0 : Constant  Value=y(3,1)
  h : Outport
  gamma : Outport  Port=2
  wires:
  Integrator/1 -> Add5/1
  Product/1 -> Integrator/1
  h0/1 -> Add5/2
  Divide/1 -> Trigonometric Function/1
  Math Function1/1 -> Add4/1
  Add5/1 -> h/1
  Trigonometric Function1/1 -> Product/2
  Add3/1 -> gamma/1, Trigonometric Function1/1
  Add4/1 -> Sqrt/1
  Trigonometric Function/1 -> Add3/1  "alpha"
  Math Function/1 -> Add4/2
  Sqrt/1 -> Product/1
  Math Function2/1 -> Add4/3
  v0/1 -> Math Function2/1
  Add/1 -> Math Function1/1, Divide/1
  u0/1 -> Add/1
  du/1 -> Add/2
  w0/1 -> Add1/2
  dw/1 -> Add1/1
  Add1/1 -> Math Function/1, Divide/2
  dtheta/1 -> Add2/1
  theta0/1 -> Add2/2
  Add2/1 -> Add3/2  "theta"

== system FINAL/Longtudinal Autopilot2/Pitch (Theta) Controller ==
  note: Pitch Controller
  theta_com(deg) : Inport
  q : Inport  Port=2
  theta : Inport  Port=3
  Elevator Saturation : Saturate  UpperLimit=25*pi/180  LowerLimit=-25*pi/180
  Kd : Gain  Gain=K_D
  Sum : Sum  Inputs=|+-
  Sum1 : Sum  Inputs=|+-
  Zero-Pole : ZeroPole  Zeros=[Z_PI]  Poles=[P_PI]  Gain=[K_PI]
  servo : TransferFcn  Numerator=[-10]  Denominator=[1 10]
  delta_elevator : Outport
  wires:
  q/1 -> Kd/1
  Zero-Pole/1 -> Sum/1
  Sum/1 -> servo/1
  theta_com(deg)/1 -> Sum1/1
  Kd/1 -> Sum/2
  theta/1 -> Sum1/2
  servo/1 -> Elevator Saturation/1
  Sum1/1 -> Zero-Pole/1
  Elevator Saturation/1 -> delta_elevator/1

== system FINAL/Longtudinal Autopilot2/Velocity Controller ==
  note: Velocity Controller
  u_com : Inport
  du : Inport  Port=2
  Engine Saturation : Saturate  UpperLimit=3*3700  LowerLimit=-1500
  Sum : Sum  Inputs=|+-
  Sum1 : Sum  Inputs=|+-
  Zero-Pole : ZeroPole  Zeros=[Z_Du]  Poles=[P_Du]  Gain=[K_Du]
  Zero-Pole1 : ZeroPole  Zeros=[Z_PIu]  Poles=[P_PIu]  Gain=[K_PIu]
  engine_timelag : TransferFcn  Numerator=[0.1]  Denominator=[1 0.1]
  servo : TransferFcn  Numerator=[10]  Denominator=[1 10]
  delta_thrust : Outport
  wires:
  u_com/1 -> Sum1/1
  Sum/1 -> servo/1
  servo/1 -> engine_timelag/1
  du/1 -> Sum1/2, Zero-Pole/1
  engine_timelag/1 -> Engine Saturation/1
  Zero-Pole/1 -> Sum/2
  Sum1/1 -> Zero-Pole1/1
  Zero-Pole1/1 -> Sum/1
  Engine Saturation/1 -> delta_thrust/1

== system FINAL/Nonlinear Model/Airframe_Model ==
  States : Inport
  delta_controls : Inport  Port=2
  Bus Selector : BusSelector  OutputSignals=u,v,w,p,q,r,Wd0t
  Constant : Constant  Value=[s0(1:6,1);0]
  Demux : Demux  Outputs=2
  Demux1 : Demux  Outputs=2
  Gain : Gain  Gain=Der(:,1:7)  Multiplication=Matrix(K*u)
  Gain3 : Gain  Gain=Der(:,8:11)  Multiplication=Matrix(K*u)
  Mux : Mux  Inputs=7
  Sum : Sum  Inputs=|+-
  Sum1 : Sum  Inputs=|++
  Sum2 : Sum  Inputs=++|
  delta_Forces : Outport
  delta_moments : Outport  Port=2
  wires:
  Constant/1 -> Sum/2
  Sum1/1 -> delta_Forces/1
  Bus Selector/6 -> Mux/6  "<r>"
  States/1 -> Bus Selector/1
  Bus Selector/7 -> Mux/7  "<Wd0t>"
  Bus Selector/5 -> Mux/5  "<q>"
  Mux/1 -> Sum/1
  Bus Selector/4 -> Mux/4  "<p>"
  Gain/1 -> Demux/1
  Sum/1 -> Gain/1
  Bus Selector/1 -> Mux/1  "<u>"
  Demux/1 -> Sum1/1
  Sum2/1 -> delta_moments/1
  Demux1/1 -> Sum1/2
  delta_controls/1 -> Gain3/1
  Gain3/1 -> Demux1/1
  Bus Selector/2 -> Mux/2  "<v>"
  Bus Selector/3 -> Mux/3  "<w>"
  Demux/2 -> Sum2/1
  Demux1/2 -> Sum2/2

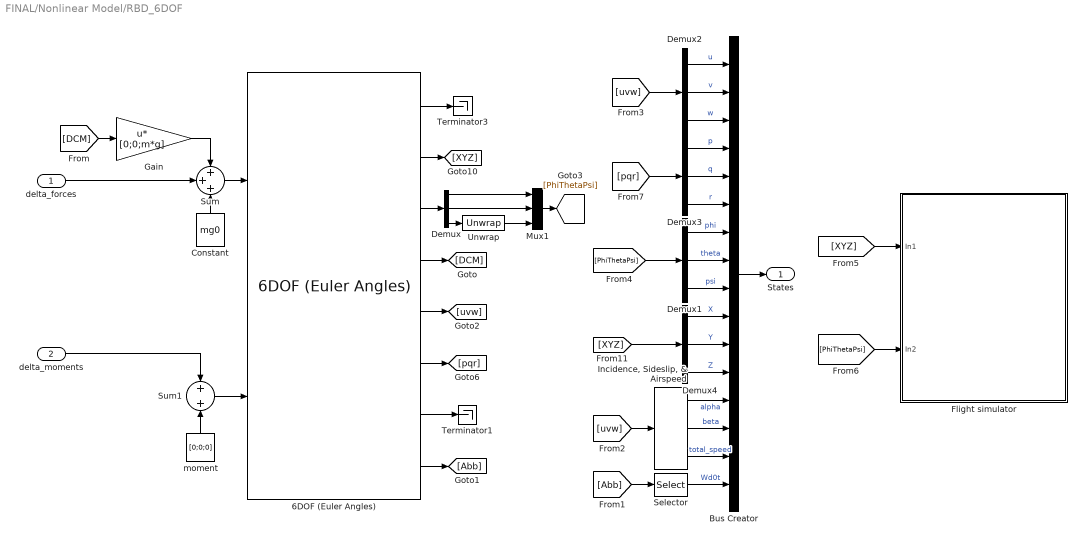
== system FINAL/Nonlinear Model/RBD_6DOF ==
  delta_forces : Inport
  delta_moments : Inport  Port=2
  6DOF (Euler Angles) : shared6dof/6DOF (Euler Angles)  units=English (Velocity in ft/s)  mtype=Fixed  rep=Euler Angles  xme_0=s0(10:12,1)  Vm_0=s0(1:3,1)  eul_0=s0(7:9,1)  pm_0=s0(4:6,1)  mass_0=m  mass_e=0.5  mass_f=2.0  inertia=I  inertia_e=eye(3)  inertia_f=2*eye(3)  k_quat=1.0  vre_flag=on  abi_flag=off  aMode=aMode  xme_statename=''  Vm_statename=''  eul_statename=''  quat_statename=''  pm_statename=''  mass_statename=''
      settings: SourceProductBaseCode=AE,PW,DR,MT,UV,VE
  Bus Creator : BusCreator  Inputs=16
  Constant : Constant  Value=mg0
  Demux{,1..4} (5 alike) : Demux  Outputs=3
  Flight simulator : Subsystem
  Gain : Gain  Gain=[0;0;m*g]  Multiplication=Matrix(u*K)
  "Incidence, Sideslip, & Airspeed" : aerolibasang/Incidence, Sideslip, & Airspeed
  Mux1 : Mux  Inputs=3
  Selector : Selector  InputPortWidth=3  IndexOptions=Index vector (dialog)  Indices=[3]  OutputSizes=1
  Sum : Sum  Inputs=+++
  Sum1 : Sum
  Terminator1 : Terminator
  Terminator3 : Terminator
  Unwrap : dspsigops/Unwrap  tol=pi  InputProcessing=Columns as channels (frame based)  running=off
  moment : Constant  Value=[0;0;0]
  States : Outport
  wires:
  Demux4/3 -> Bus Creator/12  "Z"
  6DOF (Euler Angles)/3 -> Demux/1
  6DOF (Euler Angles)/8 -> [Abb]
  Unwrap/1 -> Mux1/3
  Demux/3 -> Unwrap/1
  6DOF (Euler Angles)/7 -> Terminator1/1
  6DOF (Euler Angles)/1 -> Terminator3/1
  Sum/1 -> 6DOF (Euler Angles)/1
  Demux/1 -> Mux1/1
  6DOF (Euler Angles)/5 -> [uvw]
  Demux/2 -> Mux1/2
  Demux4/1 -> Bus Creator/10  "X"
  Demux4/2 -> Bus Creator/11  "Y"
  Constant/1 -> Sum/3
  moment/1 -> Sum1/2
  Sum1/1 -> 6DOF (Euler Angles)/2
  6DOF (Euler Angles)/4 -> [DCM]
  [Abb] -> Selector/1
  Selector/1 -> Bus Creator/16  "Wd0t"
  [uvw] -> "Incidence, Sideslip, & Airspeed"/1
  "Incidence, Sideslip, & Airspeed"/1 -> Bus Creator/13  "alpha"
  "Incidence, Sideslip, & Airspeed"/2 -> Bus Creator/14  "beta"
  "Incidence, Sideslip, & Airspeed"/3 -> Bus Creator/15  "total_speed"
  Gain/1 -> Sum/1
  [DCM] -> Gain/1
  Bus Creator/1 -> States/1
  delta_forces/1 -> Sum/2
  delta_moments/1 -> Sum1/1
  Demux1/1 -> Bus Creator/7  "phi"
  Demux1/2 -> Bus Creator/8  "theta"
  Demux1/3 -> Bus Creator/9  "psi"
  [uvw] -> Demux2/1
  Demux2/1 -> Bus Creator/1  "u"
  Demux2/2 -> Bus Creator/2  "v"
  Demux2/3 -> Bus Creator/3  "w"
  6DOF (Euler Angles)/6 -> [pqr]
  [pqr] -> Demux3/1
  Demux3/1 -> Bus Creator/4  "p"
  Demux3/2 -> Bus Creator/5  "q"
  Demux3/3 -> Bus Creator/6  "r"
  6DOF (Euler Angles)/2 -> [XYZ]
  [XYZ] -> Demux4/1
  Mux1/1 -> [PhiThetaPsi]
  [PhiThetaPsi] -> Demux1/1
  [XYZ] -> Flight simulator/1(In1)
  [PhiThetaPsi] -> Flight simulator/2(In2)

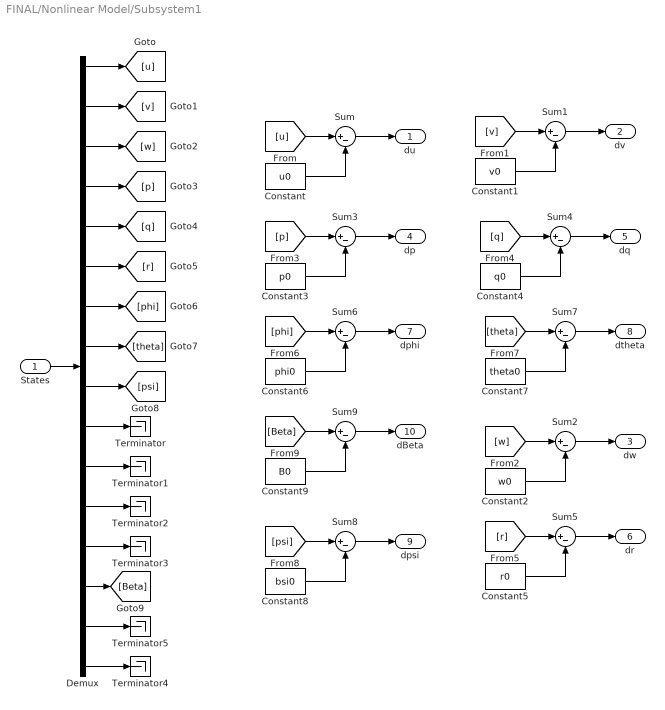
== system FINAL/Nonlinear Model/Subsystem1 ==
  States : Inport
  Constant : Constant  Value=u0
  Constant1 : Constant  Value=v0
  Constant2 : Constant  Value=w0
  Constant3 : Constant  Value=p0
  Constant4 : Constant  Value=q0
  Constant5 : Constant  Value=r0
  Constant6 : Constant  Value=phi0
  Constant7 : Constant  Value=theta0
  Constant8 : Constant  Value=bsi0
  Constant9 : Constant  Value=B0
  Demux : Demux  Outputs=16
  Sum{,1..9} (10 alike) : Sum  Inputs=|+-
  Terminator{,1..5} (6 alike) : Terminator
  du : Outport
  dv : Outport  Port=2
  dw : Outport  Port=3
  dp : Outport  Port=4
  dq : Outport  Port=5
  dr : Outport  Port=6
  dphi : Outport  Port=7
  dtheta : Outport  Port=8
  dpsi : Outport  Port=9
  dBeta : Outport  Port=10
  wires:
  States/1 -> Demux/1
  Demux/1 -> [u]
  Demux/2 -> [v]
  Demux/3 -> [w]
  Demux/4 -> [p]
  Demux/5 -> [q]
  Demux/6 -> [r]
  Demux/7 -> [phi]
  Demux/8 -> [theta]
  Demux/9 -> [psi]
  Demux/10 -> Terminator/1
  Demux/11 -> Terminator1/1
  Demux/12 -> Terminator2/1
  Demux/13 -> Terminator3/1
  Demux/15 -> Terminator5/1
  Demux/14 -> [Beta]
  [u] -> Sum/1
  Constant/1 -> Sum/2
  Sum/1 -> du/1
  [v] -> Sum1/1
  Sum1/1 -> dv/1
  Constant1/1 -> Sum1/2
  [w] -> Sum2/1
  Sum2/1 -> dw/1
  Constant2/1 -> Sum2/2
  [p] -> Sum3/1
  Sum3/1 -> dp/1
  Constant3/1 -> Sum3/2
  [q] -> Sum4/1
  Sum4/1 -> dq/1
  Constant4/1 -> Sum4/2
  [r] -> Sum5/1
  Sum5/1 -> dr/1
  Constant5/1 -> Sum5/2
  [phi] -> Sum6/1
  Sum6/1 -> dphi/1
  [psi] -> Sum8/1
  Constant8/1 -> Sum8/2
  Sum7/1 -> dtheta/1
  Sum8/1 -> dpsi/1
  Constant7/1 -> Sum7/2
  [theta] -> Sum7/1
  Constant6/1 -> Sum6/2
  Constant9/1 -> Sum9/2
  [Beta] -> Sum9/1
  Sum9/1 -> dBeta/1
  Demux/16 -> Terminator4/1

== system FINAL/Nonlinear Model/RBD_6DOF/Flight simulator ==
  In1 : Inport
  In2 : Inport  Port=2
  Demux : Demux  Outputs=2
  Demux1 : Demux  Outputs=3
  Flat Earth to LLA : aerolibtransform2/Flat Earth to LLA  units=Metric (MKS)  ptype=Earth (WGS84)  F=1/298.257223563  R=6378137  refPosPort=off  LL0=[0 10]  psi=0
  FlightGear Preconfigured 6DoF Animation : aerolibfltsims/FlightGear Preconfigured 6DoF Animation  xFlightGearVersion=v2019.1  DestinationIpAddress=127.0.0.1  DestinationPort=5502  SampleTime=dt  packetVersion=24
  Generate Run Script : aerolibfltsims/Generate Run Script  Architecture=Default  dataFlow=Send  GeometryModelName=Lockheed1049h  AirportId=KSFO  RunwayId=10L  InitialAltitude=7224  InitialHeading=113  OffsetDistance=4.72  OffsetAzimuth=0  InstallScenery=off  DisableShaders=on  OriginAddress=127.0.0.1  DestinationPort=5502  OriginPort=5505  LocalAddress=127.0.0.1  OutputFileName=Simulator.bat  FlightGearBaseDirectory=C:\Program Files\FlightGear 2020.3
  Ground : Ground
  Mux : Mux
  Mux1 : Mux  Inputs=3
  wires:
  Ground/1 -> Flat Earth to LLA/2
  Flat Earth to LLA/1 -> Demux/1
  Demux/1 -> Mux/2
  Demux/2 -> Mux/1
  Flat Earth to LLA/2 -> Mux/3
  Mux/1 -> FlightGear Preconfigured 6DoF Animation/1
  In2/1 -> Mux/4
  In1/1 -> Demux1/1
  Mux1/1 -> Flat Earth to LLA/1
  Demux1/1 -> Mux1/1
  Demux1/2 -> Mux1/2
  Demux1/3 -> Mux1/3
